simulink model "Maglev_sim_1"  (R2024b)
settings: Solver=ode23tb  StartTime=0.0  StopTime=15  MaxStep=1e-3  RelTol=1e-3
undefined symbols (not defined in the file): A, A0, A0_obv, Aa_obv, Adj, B, B0, B0_obv, Ba_obv, c, C, C0, C0_obv, Ca_obv, D0, D0_obv, Da_obv, G, K, K0
libraries: simulink x2
settings Model: Creator=coron  LastModifiedBy=guide

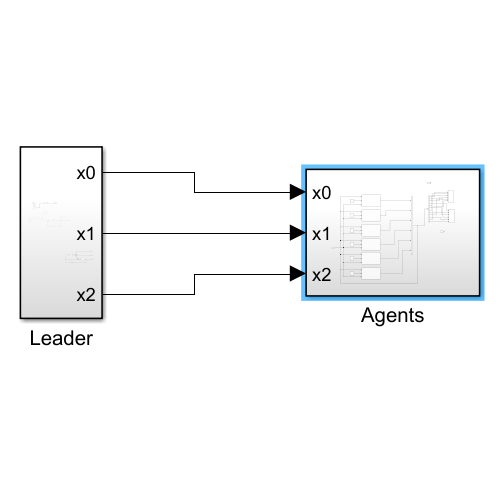
[thumbnail: Simulink's stored preview of the top-level diagram]
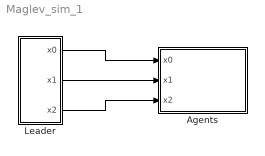
== system Maglev_sim_1 ==
  Agents : Subsystem
  Leader : Subsystem
  wires:
  Leader/1(x0) -> Agents/1(x0)
  Leader/2(x1) -> Agents/2(x1)
  Leader/3(x2) -> Agents/3(x2)

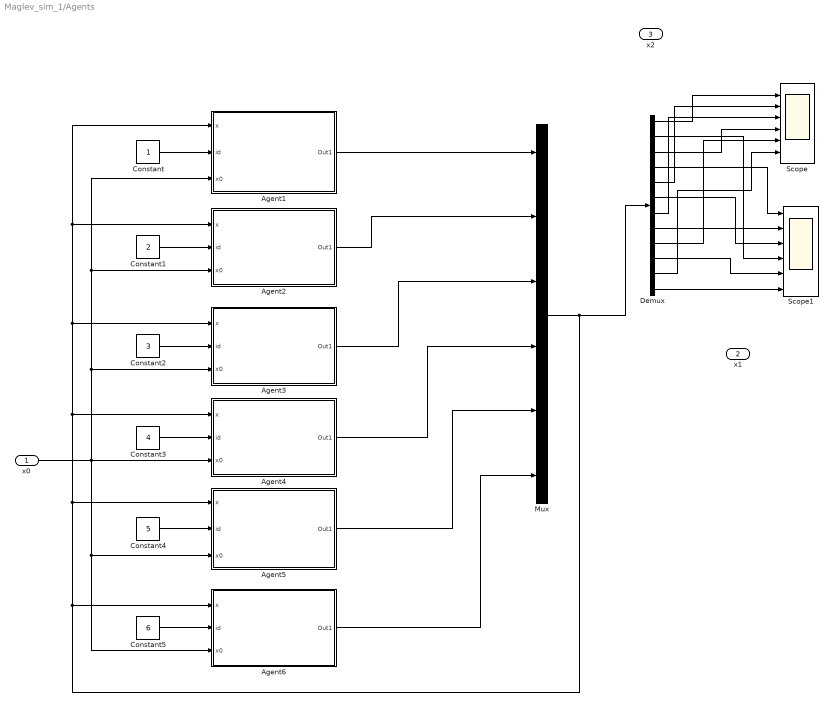
== system Maglev_sim_1/Agents ==
  x0 : Inport
  x1 : Inport  Port=2
  x2 : Inport  Port=3
  Agent1 : Subsystem
  Agent2 : Subsystem
  Agent3 : Subsystem
  Agent4 : Subsystem
  Agent5 : Subsystem
  Agent6 : Subsystem
  Constant : Constant
  Constant1 : Constant  Value=2
  Constant2 : Constant  Value=3
  Constant3 : Constant  Value=4
  Constant4 : Constant  Value=5
  Constant5 : Constant  Value=6
  Demux : Demux  Outputs=12
  Mux : Mux  Inputs=6
  Scope : Scope  NumInputPorts=6
  Scope1 : Scope  NumInputPorts=6
  wires:
  Constant1/1 -> Agent2/2(id)
  Agent2/1(Out1) -> Mux/2
  Agent5/1(Out1) -> Mux/5
  x0/1 -> Agent6/3(x0), Agent5/3(x0), Agent1/3(x0), Agent2/3(x0), Agent3/3(x0), Agent4/3(x0)
  Mux/1 -> Agent2/1(x), Agent1/1(x), Agent3/1(x), Agent4/1(x), Agent5/1(x), Agent6/1(x), Demux/1
  Constant2/1 -> Agent3/2(id)
  Agent3/1(Out1) -> Mux/3
  Constant3/1 -> Agent4/2(id)
  Agent6/1(Out1) -> Mux/6
  Constant4/1 -> Agent5/2(id)
  Constant5/1 -> Agent6/2(id)
  Constant/1 -> Agent1/2(id)
  Agent1/1(Out1) -> Mux/1
  Agent4/1(Out1) -> Mux/4
  Demux/1 -> Scope/1
  Demux/2 -> Scope1/4
  Demux/3 -> Scope/4
  Demux/4 -> Scope1/1
  Demux/5 -> Scope/2
  Demux/6 -> Scope1/3
  Demux/7 -> Scope/3
  Demux/8 -> Scope1/2
  Demux/9 -> Scope/5
  Demux/10 -> Scope1/5
  Demux/11 -> Scope/6
  Demux/12 -> Scope1/6

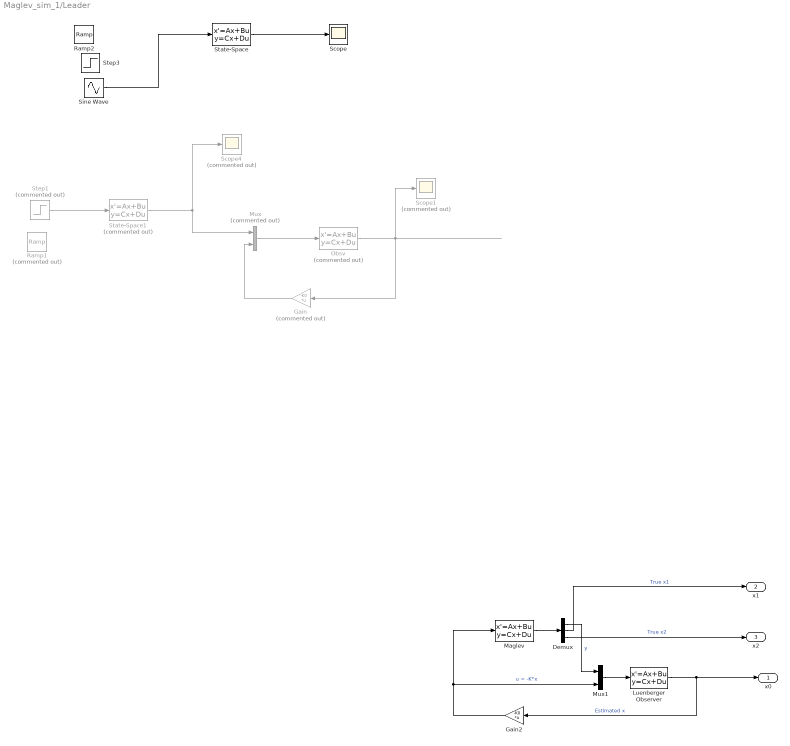
== system Maglev_sim_1/Leader ==
  Demux : Demux  Outputs=3
  Gain : Gain  Commented=on  Gain=-K0  Multiplication=Matrix(K*u) (u vector)
  Gain2 : Gain  Gain=-K0  Multiplication=Matrix(K*u)
  Luenberger Observer : StateSpace  A=A0_obv  B=B0_obv  C=C0_obv  D=D0_obv  InitialCondition=0
  Maglev : StateSpace  A=A0  B=B0  C=C0  D=D0  InitialCondition=[0 10]'
  Mux : Mux  Commented=on  Inputs=2
  Mux1 : Mux  Inputs=2
  Obsv : StateSpace  Commented=on  A=A0_obv  B=B0_obv  C=C0_obv  D=D0_obv  InitialCondition=0
  Ramp1 : simulink/Sources/Ramp  Commented=on  slope=-1  start=0  InitialOutput=0
  Ramp2 : simulink/Sources/Ramp  slope=-1  start=0  InitialOutput=0
  Scope : Scope
  Scope1 : Scope  Commented=on
  Scope4 : Scope  Commented=on
  Sine Wave : Sin  SampleTime=0
  State-Space : StateSpace  A=A0-B*K0  B=B0  C=eye(2)  D=zeros(2,1)  InitialCondition=0
  State-Space1 : StateSpace  Commented=on  A=A0-B*K0  B=B0  C=C0  D=D0  InitialCondition=0
  Step1 : Step  Commented=on  After=-1  SampleTime=0
  Step3 : Step  After=-1  SampleTime=0
  x0 : Outport
  x1 : Outport  Port=2
  x2 : Outport  Port=3
  wires:
  Gain/1 -> Mux/2
  State-Space1/1 -> Mux/1, Scope4/1
  Obsv/1 -> Scope1/1, Gain/1
  Step1/1 -> State-Space1/1
  State-Space/1 -> Scope/1
  Mux/1 -> Obsv/1
  Sine Wave/1 -> State-Space/1
  Mux1/1 -> Luenberger Observer/1
  Gain2/1 -> Maglev/1, Mux1/2  "u = -K*x"
  Luenberger Observer/1 -> x0/1, Gain2/1  "Estimated x"
  Maglev/1 -> Demux/1
  Demux/2 -> x1/1  "True x1"
  Demux/1 -> Mux1/1  "y"
  Demux/3 -> x2/1  "True x2"

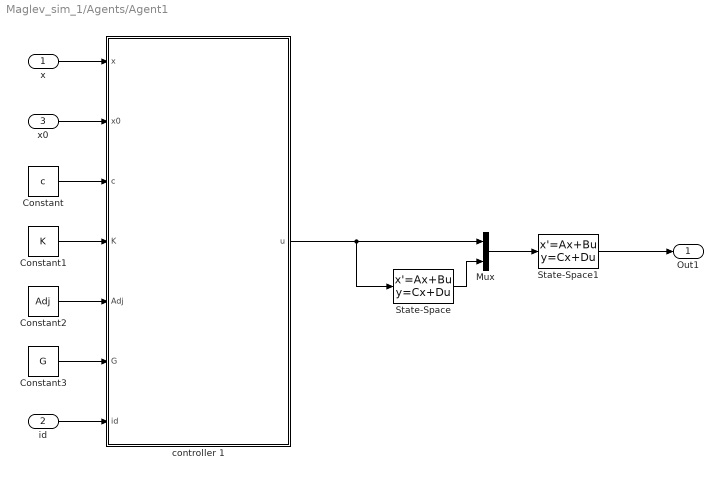
== system Maglev_sim_1/Agents/Agent1 ==
  x : Inport
  id : Inport  Port=2
  x0 : Inport  Port=3
  Constant : Constant  Value=c
  Constant1 : Constant  Value=K  VectorParams1D=off
  Constant2 : Constant  Value=Adj
  Constant3 : Constant  Value=G
  Mux : Mux  Inputs=2
  State-Space : StateSpace  A=(A-B*K0)  B=B  C=C  D=0  InitialCondition=0
  State-Space1 : StateSpace  A=Aa_obv  B=Ba_obv  C=Ca_obv  D=Da_obv  InitialCondition=0
  controller 1 : MATLAB Function  TreatAsAtomicUnit=on
  Out1 : Outport
  wires:
  x/1 -> controller 1/1(x)
  Constant/1 -> controller 1/3(c)
  Constant1/1 -> controller 1/4(K)
  Constant2/1 -> controller 1/5(Adj)
  Constant3/1 -> controller 1/6(G)
  id/1 -> controller 1/7(id)
  controller 1/1(u) -> Mux/1, State-Space/1
  x0/1 -> controller 1/2(x0)
  State-Space1/1 -> Out1/1
  Mux/1 -> State-Space1/1
  State-Space/1 -> Mux/2

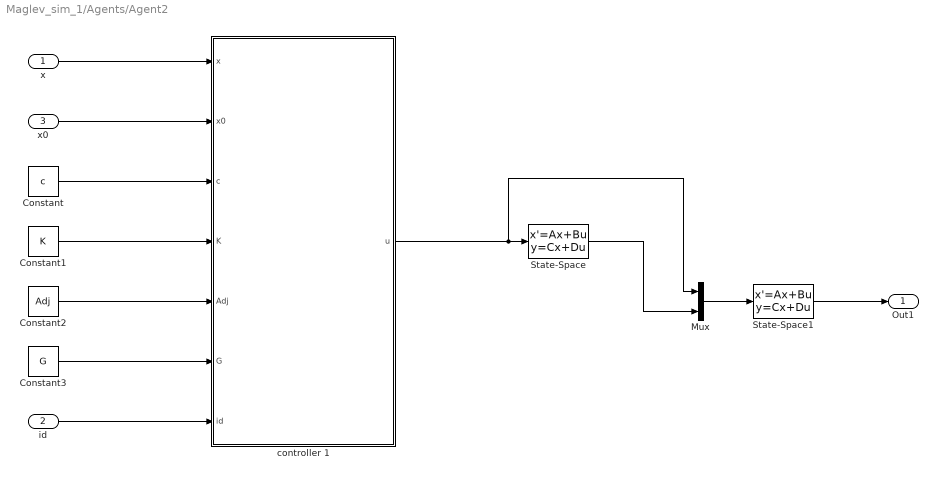
== system Maglev_sim_1/Agents/Agent2 ==
  x : Inport
  id : Inport  Port=2
  x0 : Inport  Port=3
  Constant : Constant  Value=c
  Constant1 : Constant  Value=K  VectorParams1D=off
  Constant2 : Constant  Value=Adj
  Constant3 : Constant  Value=G
  Mux : Mux  Inputs=2
  State-Space : StateSpace  A=(A-B*K0)  B=B  C=C  D=0  InitialCondition=0
  State-Space1 : StateSpace  A=Aa_obv  B=Ba_obv  C=Ca_obv  D=Da_obv  InitialCondition=0
  controller 1 : MATLAB Function  TreatAsAtomicUnit=on
  Out1 : Outport
  wires:
  State-Space1/1 -> Out1/1
  Mux/1 -> State-Space1/1
  id/1 -> controller 1/7(id)
  Constant2/1 -> controller 1/5(Adj)
  State-Space/1 -> Mux/2
  Constant1/1 -> controller 1/4(K)
  controller 1/1(u) -> Mux/1, State-Space/1
  Constant3/1 -> controller 1/6(G)
  x0/1 -> controller 1/2(x0)
  Constant/1 -> controller 1/3(c)
  x/1 -> controller 1/1(x)

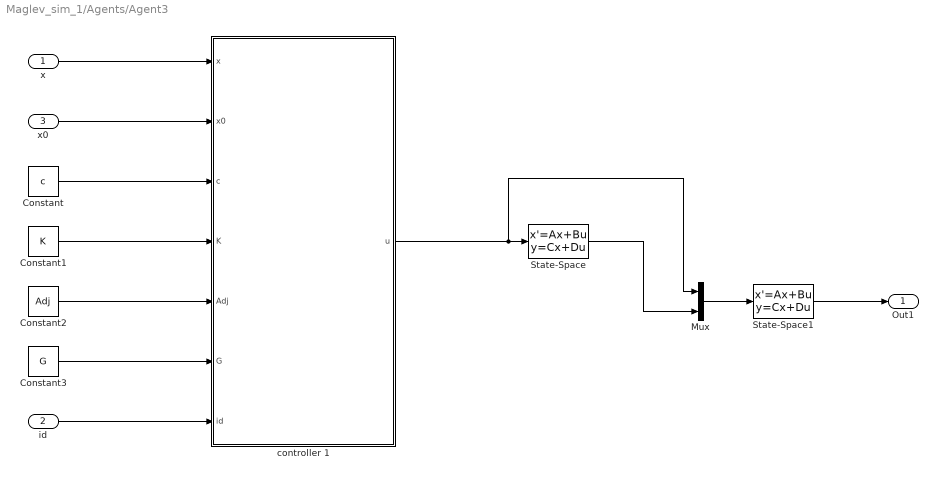
== system Maglev_sim_1/Agents/Agent3 ==
  x : Inport
  id : Inport  Port=2
  x0 : Inport  Port=3
  Constant : Constant  Value=c
  Constant1 : Constant  Value=K  VectorParams1D=off
  Constant2 : Constant  Value=Adj
  Constant3 : Constant  Value=G
  Mux : Mux  Inputs=2
  State-Space : StateSpace  A=(A-B*K0)  B=B  C=C  D=0  InitialCondition=0
  State-Space1 : StateSpace  A=Aa_obv  B=Ba_obv  C=Ca_obv  D=Da_obv  InitialCondition=0
  controller 1 : MATLAB Function  TreatAsAtomicUnit=on
  Out1 : Outport
  wires:
  State-Space1/1 -> Out1/1
  Mux/1 -> State-Space1/1
  id/1 -> controller 1/7(id)
  Constant2/1 -> controller 1/5(Adj)
  State-Space/1 -> Mux/2
  Constant1/1 -> controller 1/4(K)
  controller 1/1(u) -> Mux/1, State-Space/1
  Constant3/1 -> controller 1/6(G)
  x0/1 -> controller 1/2(x0)
  Constant/1 -> controller 1/3(c)
  x/1 -> controller 1/1(x)

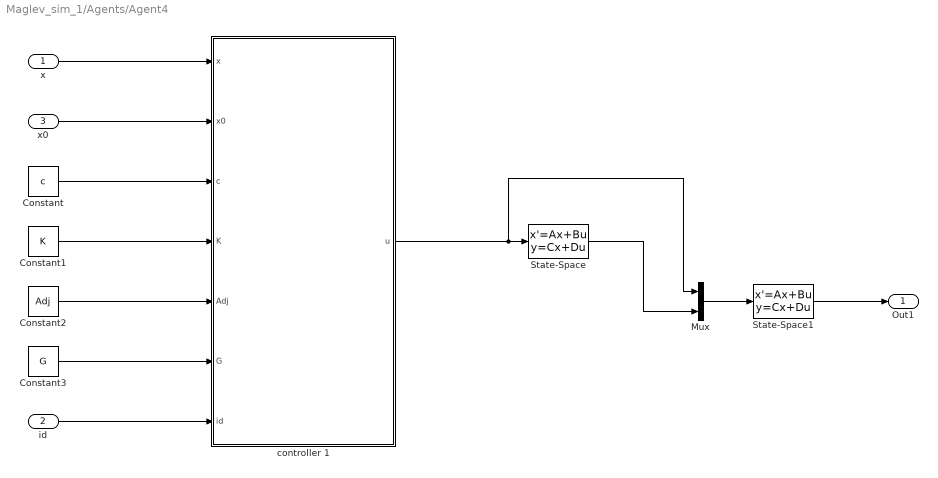
== system Maglev_sim_1/Agents/Agent4 ==
  x : Inport
  id : Inport  Port=2
  x0 : Inport  Port=3
  Constant : Constant  Value=c
  Constant1 : Constant  Value=K  VectorParams1D=off
  Constant2 : Constant  Value=Adj
  Constant3 : Constant  Value=G
  Mux : Mux  Inputs=2
  State-Space : StateSpace  A=(A-B*K0)  B=B  C=C  D=0  InitialCondition=0
  State-Space1 : StateSpace  A=Aa_obv  B=Ba_obv  C=Ca_obv  D=Da_obv  InitialCondition=0
  controller 1 : MATLAB Function  TreatAsAtomicUnit=on
  Out1 : Outport
  wires:
  State-Space1/1 -> Out1/1
  Mux/1 -> State-Space1/1
  id/1 -> controller 1/7(id)
  Constant2/1 -> controller 1/5(Adj)
  State-Space/1 -> Mux/2
  Constant1/1 -> controller 1/4(K)
  controller 1/1(u) -> Mux/1, State-Space/1
  Constant3/1 -> controller 1/6(G)
  x0/1 -> controller 1/2(x0)
  Constant/1 -> controller 1/3(c)
  x/1 -> controller 1/1(x)

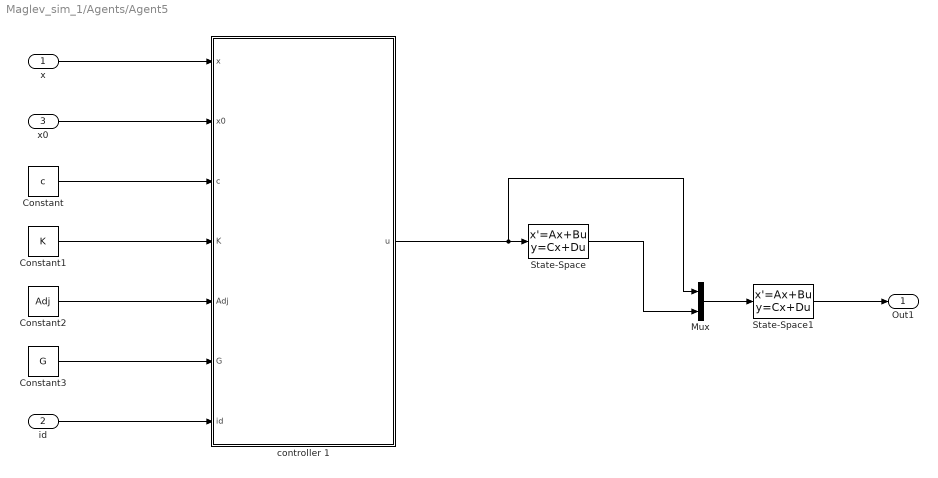
== system Maglev_sim_1/Agents/Agent5 ==
  x : Inport
  id : Inport  Port=2
  x0 : Inport  Port=3
  Constant : Constant  Value=c
  Constant1 : Constant  Value=K  VectorParams1D=off
  Constant2 : Constant  Value=Adj
  Constant3 : Constant  Value=G
  Mux : Mux  Inputs=2
  State-Space : StateSpace  A=(A-B*K0)  B=B  C=C  D=0  InitialCondition=0
  State-Space1 : StateSpace  A=Aa_obv  B=Ba_obv  C=Ca_obv  D=Da_obv  InitialCondition=0
  controller 1 : MATLAB Function  TreatAsAtomicUnit=on
  Out1 : Outport
  wires:
  State-Space1/1 -> Out1/1
  Mux/1 -> State-Space1/1
  id/1 -> controller 1/7(id)
  Constant2/1 -> controller 1/5(Adj)
  State-Space/1 -> Mux/2
  Constant1/1 -> controller 1/4(K)
  controller 1/1(u) -> Mux/1, State-Space/1
  Constant3/1 -> controller 1/6(G)
  x0/1 -> controller 1/2(x0)
  Constant/1 -> controller 1/3(c)
  x/1 -> controller 1/1(x)

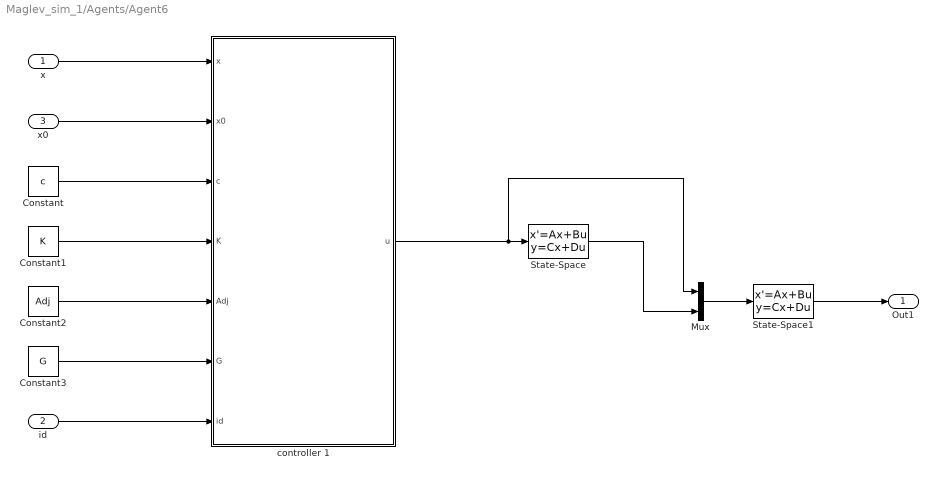
== system Maglev_sim_1/Agents/Agent6 ==
  x : Inport
  id : Inport  Port=2
  x0 : Inport  Port=3
  Constant : Constant  Value=c
  Constant1 : Constant  Value=K  VectorParams1D=off
  Constant2 : Constant  Value=Adj
  Constant3 : Constant  Value=G
  Mux : Mux  Inputs=2
  State-Space : StateSpace  A=(A-B*K0)  B=B  C=C  D=0  InitialCondition=0
  State-Space1 : StateSpace  A=Aa_obv  B=Ba_obv  C=Ca_obv  D=Da_obv  InitialCondition=0
  controller 1 : MATLAB Function  TreatAsAtomicUnit=on
  Out1 : Outport
  wires:
  State-Space1/1 -> Out1/1
  Mux/1 -> State-Space1/1
  id/1 -> controller 1/7(id)
  Constant2/1 -> controller 1/5(Adj)
  State-Space/1 -> Mux/2
  Constant1/1 -> controller 1/4(K)
  controller 1/1(u) -> Mux/1, State-Space/1
  Constant3/1 -> controller 1/6(G)
  x0/1 -> controller 1/2(x0)
  Constant/1 -> controller 1/3(c)
  x/1 -> controller 1/1(x)

== matlab function Maglev_sim_1/Agents/Agent1/controller 1 ==
  data: x input; x0 input; u output; c input; K input; Adj input; G input; id input
function u = controller(x,x0,c,K,Adj,G,id)


pairs = reshape(x, 2, [])';

error = zeros(2,1);

for j = 1:6
    error = error + Adj(id,j)*(pairs(j,:)'-pairs(id,:)')+G(id)*(x0 - pairs(id,:)');
end

u=c*K*error;

== matlab function Maglev_sim_1/Agents/Agent2/controller 1 ==
  data: x input; x0 input; u output; c input; K input; Adj input; G input; id input
function u = controller(x,x0,c,K,Adj,G,id)


pairs = reshape(x, 2, [])';

error = zeros(2,1);

for j = 1:6
    error = error + Adj(id,j)*(pairs(j,:)'-pairs(id,:)')+G(id)*(x0 - pairs(id,:)');
end

u=c*K*error;

== matlab function Maglev_sim_1/Agents/Agent6/controller 1 ==
  data: x input; x0 input; u output; c input; K input; Adj input; G input; id input
function u = controller(x,x0,c,K,Adj,G,id)


pairs = reshape(x, 2, [])';

error = zeros(2,1);

for j = 1:6
    error = error + Adj(id,j)*(pairs(j,:)'-pairs(id,:)')+G(id)*(x0 - pairs(id,:)');
end

u=c*K*error;

== matlab function Maglev_sim_1/Agents/Agent3/controller 1 ==
  data: x input; x0 input; u output; c input; K input; Adj input; G input; id input
function u = controller(x,x0,c,K,Adj,G,id)


pairs = reshape(x, 2, [])';

error = zeros(2,1);

for j = 1:6
    error = error + Adj(id,j)*(pairs(j,:)'-pairs(id,:)')+G(id)*(x0 - pairs(id,:)');
end

u=c*K*error;

== matlab function Maglev_sim_1/Agents/Agent4/controller 1 ==
  data: x input; x0 input; u output; c input; K input; Adj input; G input; id input
function u = controller(x,x0,c,K,Adj,G,id)


pairs = reshape(x, 2, [])';

error = zeros(2,1);

for j = 1:6
    error = error + Adj(id,j)*(pairs(j,:)'-pairs(id,:)')+G(id)*(x0 - pairs(id,:)');
end

u=c*K*error;

== matlab function Maglev_sim_1/Agents/Agent5/controller 1 ==
  data: x input; x0 input; u output; c input; K input; Adj input; G input; id input
function u = controller(x,x0,c,K,Adj,G,id)


pairs = reshape(x, 2, [])';

error = zeros(2,1);

for j = 1:6
    error = error + Adj(id,j)*(pairs(j,:)'-pairs(id,:)')+G(id)*(x0 - pairs(id,:)');
end

u=c*K*error;
